simulink model "Prob5"  (R2020b)
settings: Solver=VariableStepAuto  StartTime=0.0  StopTime=10.0  RelTol=1e-3
model workspace (MAT data in the model file):
  C = Simulink.Parameter
  C.Value = 1e-05
  C.DataType = 'auto'
  C.Dimensions = [1 1]
  R = Simulink.Parameter
  R.Value = 10
  R.DataType = 'auto'
  R.Dimensions = [1 1]
settings Model: Creator=shoun  LastModifiedBy=shoun

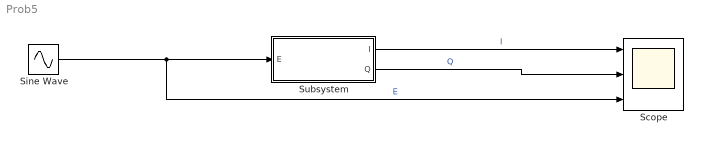
== system Prob5 ==
  Scope : Scope  NumInputPorts=3
  Sine Wave : Sin  SampleTime=0
  Subsystem : Subsystem  mask{C=10^-5, R=10}
  wires:
  Sine Wave/1 -> Scope/3, Subsystem/1(E)  "E"
  Subsystem/1(I) -> Scope/1  "I"
  Subsystem/2(Q) -> Scope/2  "Q"

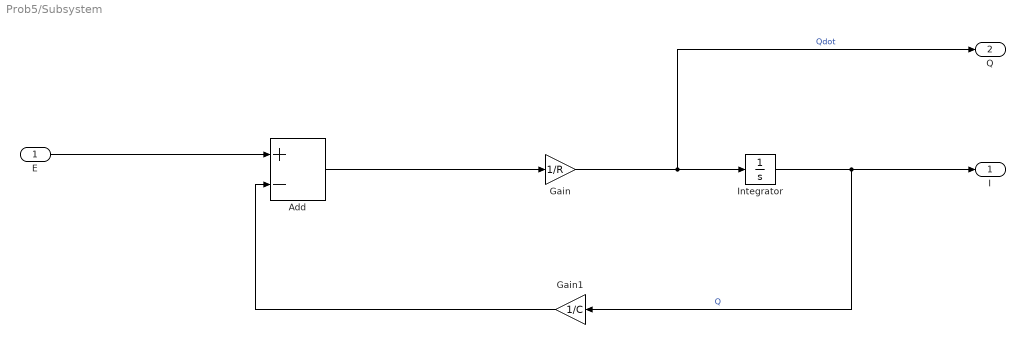
== system Prob5/Subsystem ==
  E : Inport
  Add : Sum  Inputs=+-
  Gain : Gain  Gain=1/R
  Gain1 : Gain  Gain=1/C
  Integrator : Integrator
  I : Outport
  Q : Outport  Port=2
  wires:
  Add/1 -> Gain/1
  Gain/1 -> Q/1, Integrator/1  "Qdot"
  Integrator/1 -> Gain1/1, I/1  "Q"
  E/1 -> Add/1
  Gain1/1 -> Add/2
